simulink model "notch_filter_config_set"  (R2023a)
settings: configuration reference "config" (kept outside this file)
model workspace (MAT data in the model file):
  damp = Simulink.Parameter
  damp.Value = 10
  damp.DataType = 'double'
  damp.Complexity = 'real'
  damp.Dimensions = [1 1]
  dt = Simulink.Parameter
  dt.Value = 0.0001
  dt.DataType = 'double'
  dt.Complexity = 'real'
  dt.Dimensions = [1 1]
  freq = Simulink.Parameter
  freq.Value = 439
  freq.DataType = 'double'
  freq.Complexity = 'real'
  freq.Dimensions = [1 1]
  gmin = Simulink.Parameter
  gmin.Value = 100
  gmin.DataType = 'double'
  gmin.Complexity = 'real'
  gmin.Dimensions = [1 1]
undefined symbols (not defined in the file): u0, u1, u2, y0, y1
settings Model: DataDictionary=model_config.sldd  ParameterArgumentNames=damp,dt,freq,gmin  Creator=GQR  LastModifiedBy=Administrator
settings ConfigSetRef: SourceName=config

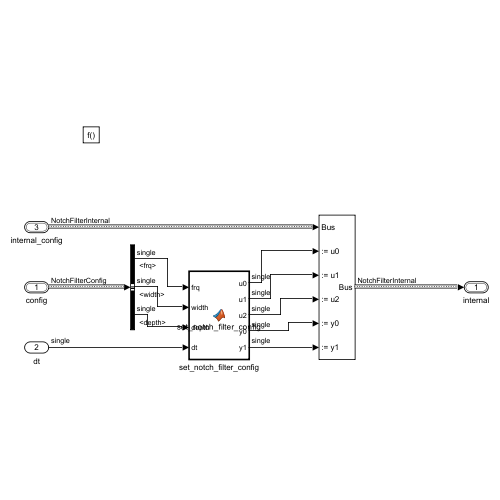
[thumbnail: Simulink's stored preview of the top-level diagram]
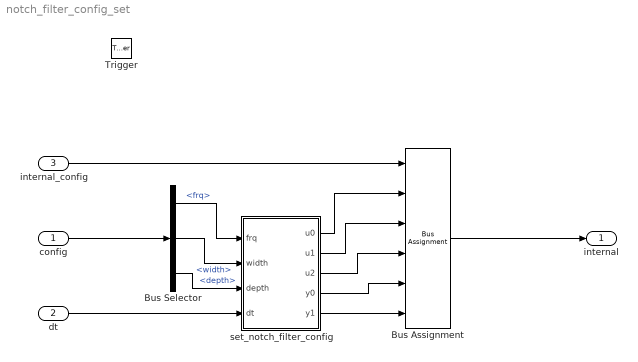
== system notch_filter_config_set ==
  config : Inport  OutDataTypeStr=Bus: NotchFilterConfig  BusOutputAsStruct=on
  dt : Inport  Port=2  OutDataTypeStr=single
  internal_config : Inport  Port=3  OutDataTypeStr=Bus: NotchFilterInternal  BusOutputAsStruct=on
  Trigger : TriggerPort  TriggerType=function-call  VariantControl=(inherit)  PortDimensions=1
  Bus Assignment : BusAssignment  AssignedSignals=u0,u1,u2,y0,y1
  Bus Selector : BusSelector  OutputSignals=frq,width,depth
  set_notch_filter_config : MATLAB Function  TreatAsAtomicUnit=on
  internal : Outport  OutDataTypeStr=Bus: NotchFilterInternal  BusOutputAsStruct=on
  wires:
  set_notch_filter_config/1(u0) -> Bus Assignment/2
  config/1 -> Bus Selector/1
  internal_config/1 -> Bus Assignment/1
  Bus Selector/1 -> set_notch_filter_config/1(frq)  "<frq>"
  Bus Selector/2 -> set_notch_filter_config/2(width)  "<width>"
  set_notch_filter_config/2(u1) -> Bus Assignment/3
  Bus Selector/3 -> set_notch_filter_config/3(depth)  "<depth>"
  dt/1 -> set_notch_filter_config/4(dt)
  set_notch_filter_config/3(u2) -> Bus Assignment/4
  set_notch_filter_config/4(y0) -> Bus Assignment/5
  set_notch_filter_config/5(y1) -> Bus Assignment/6
  Bus Assignment/1 -> internal/1

== matlab function notch_filter_config_set/set_notch_filter_config ==
  data: frq input; width input; depth input; dt input; u0 output; u1 output; u2 output; y0 output; y1 output
function [u0, u1, u2, y0, y1] = set_notch_filter_config(frq, width, depth, dt)

num = uint8(6);  %6组滤波器
b0 = single(0);
b1 = single(0);
b2 = single(0);

u2 = single(zeros(num, 1));
u0 = single(zeros(num, 1));
u1 = single(zeros(num, 1));
y0 = single(zeros(num, 1));
y1 = single(zeros(num, 1));

for i=1:1:num 
    if frq(i) < single(0.0001)  % 频率设置为0.0fHZ  表示滤波器不生效 frq 必须 >=0
        u2(i) = single(1.0);
        u0(i) = single(0.0);
        u1(i) = single(0.0);
        y0(i) = single(0.0);
        y1(i) = single(0.0);
    else
        b0 = frq(i) * single(2.0) * pi;
        b2 = width(i) * single(2.0) * pi;
        b1 = depth(i) * b2;

        u2(i) = (dt + 2*b1/(b0*b0) + 4/(dt*b0*b0)) / (dt + 2*b2/(b0*b0) + 4/(dt*b0*b0));
        u1(i) = (2*dt - 8/(dt*b0*b0)) / (dt + 2*b2/(b0*b0) + 4/(dt*b0*b0));
        u0(i) = (dt - 2*b1/(b0*b0) + 4/(dt*b0*b0)) / (dt + 2*b2/(b0*b0) + 4/(dt*b0*b0));
        
        y1(i) = -(2*dt - 8/(dt*b0*b0)) / (dt + 2*b2/(b0*b0) + 4/(dt*b0*b0));
        y0(i) = -(dt - 2*b2/(b0*b0) + 4/(dt*b0*b0)) / (dt + 2*b2/(b0*b0) + 4/(dt*b0*b0));
    end
end


end
